simulink model "E2_Simulink"  (R2023a)
settings: Solver=VariableStepAuto  StartTime=0.0  StopTime=0.01  RelTol=1e-3
values from neighbouring files (symbols this model uses):
  c = 10e-6    (= 1e-05)    [E2_Parametros.m]
  l = 2e-3    (= 0.002)    [E2_Parametros.m]
  r = 10    [E2_Parametros.m]
  vin = 32    [E2_Parametros.m]
settings Model: Creator=mluser  LastModifiedBy=mluser

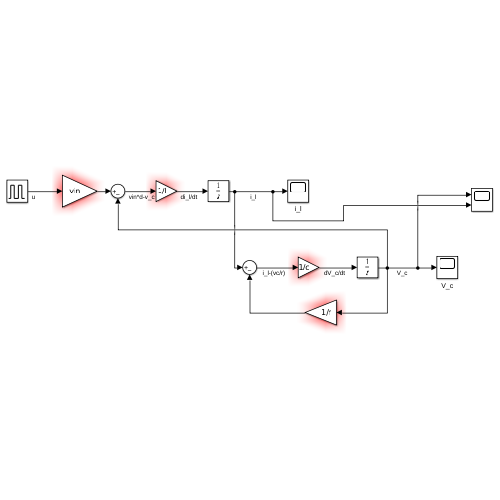
[thumbnail: Simulink's stored preview of the top-level diagram]
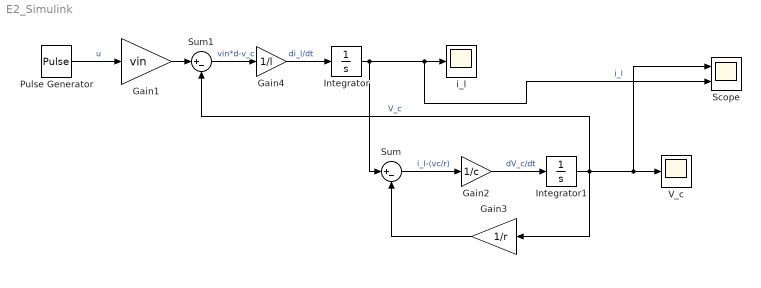
== system E2_Simulink ==
  Gain1 : Gain  Gain=vin
  Gain2 : Gain  Gain=1/c
  Gain3 : Gain  Gain=1/r
  Gain4 : Gain  Gain=1/l
  Integrator : Integrator
  Integrator1 : Integrator
  Pulse Generator : DiscretePulseGenerator  PulseType=Time based  Period=1/100e3  PulseWidth=40
  Scope : Scope  NumInputPorts=2
  Sum : Sum  Inputs=|+-
  Sum1 : Sum  Inputs=|+-
  V_c : Scope
  i_l : Scope
  wires:
  Pulse Generator/1 -> Gain1/1  "u"
  Integrator/1 -> Scope/2, i_l/1, Sum/1  "i_l"
  Integrator1/1 -> Sum1/2, Gain3/1, Scope/1, V_c/1  "V_c"
  Sum/1 -> Gain2/1  "i_l-(vc/r)"
  Gain3/1 -> Sum/2
  Gain1/1 -> Sum1/1
  Gain4/1 -> Integrator/1  "di_l/dt"
  Sum1/1 -> Gain4/1  "vin*d-v_c"
  Gain2/1 -> Integrator1/1  "dV_c/dt"
